simulink model "pompev3"  (R2021a)
settings: Solver=ode15s  StartTime=0.0  StopTime=500.0  FixedStep=0.1  RelTol=1e-3  EnableMultiTasking=on
settings Model: Creator=M1  LastModifiedBy=M1
settings SolverCC: AlgebraicLoopSolver=TrustRegion  AutoInsertRateTranBlk=on
settings DataIOCC: LimitDataPoints=on
settings OptimizationCC: LifeSpan=inf
settings DebuggingCC: AllowSymbolicDim=off  SFUnexpectedBacktrackingDiag=warning  SFNoUnconditionalDefaultTransitionDiag=warning  SFExecutionAtInitializationDiag=none  ArithmeticOperatorsInVariantConditions=warning
settings SFSimCC: SimUseLocalCustomCode=off  CustomCodeUndefinedFunction=UseInterfaceOnly
settings RTWCC: RTWUseLocalCustomCode=off
settings CodeAppCC: StateflowObjectComments=on
settings GRTTargetCC: TargetLangStandard=C89/C90 (ANSI)
settings ConfigComp: CovMetricSettings=dw  CovSaveCumulativeToWorkspaceVar=on  CovSaveSingleToWorkspaceVar=on  CovExternalEMLEnable=off  CovSFcnEnable=off

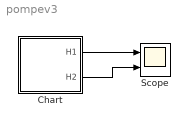
== system pompev3 ==
  Chart : Stateflow chart  TreatAsAtomicUnit=on
  Scope : Scope  NumInputPorts=2
  wires:
  Chart/1(H1) -> Scope/1
  Chart/2(H2) -> Scope/2

== stateflow chart pompev3/Chart ==
  settings: updateMethod=CONTINUOUS
  state Reservoir [parallel]
    settings: executionOrder=1
    state mode_1
      during :
      H1_dot = [(1/S)*(Qp-a*H1(1)^(1/2)-a*sign(H1(1) - H2(1))*abs(H1(1) - H2(1))^(1/2));
      - (2*H1(2))/(385*H1(1)^(1/2)) - (2*sign(H1(1) - H2(1))^2*(H1(2) - H2(2)))/(385*abs(H1(1) - H2(1))^(1/2)) - (8*abs(H1(1) - H2(1))^(1/2)*dirac*(H1(2) - H2(2)))/385];
      H2_dot = [(1/S)*a*sign(H1(1)-H2(1))*abs(H1(1)-H2(1))^(1/2);
      (2*sign(H1(1) - H2(1))^2*(H1(2) - H2(2)))/(385*abs(H1(1) - H2(1))^(1/2)) + (8*abs(H1(1) - H2(1))^(1/2)*dirac*(H1(2) - H2(2)))/385];
    note: modes 1 et 2 sont les états du réservoirs lorsque la vanne V4 est fermée
        | modes 3 et 4 sont les états du réservoirs lorsque la vanne V4 est ouverte
        | les équations se basent sur les écouelemnts de Toricelli
    state mode_2
      during :
      H1_dot = [(1/S)*(Qp-a*H1(1)^(1/2)-a*sign(H1(1) - H2(1))*abs(H1(1) - H2(1))^(1/2)-a*sign(H1(1) - H2(1))*abs(H1(1)-0.5)^(1/2));
      - (2*H1(2))/(385*H1(1)^(1/2)) - (2*sign(H1(1) - H2(1))^2*(H1(2) - H2(2)))/(385*abs(H1(1) - H2(1))^(1/2)) - (8*abs(H1(1) - 1/2)^(1/2)*dirac*(H1(2) - H2(2)))/385- (8*abs(H1(1) - H2(1))^(1/2)*dirac*(H1(2) - H2(2)))/385 - (2*sign(H1(1) - 1/2)*sign(H1(1) - H2(1))*H1(2))/(385*abs(H1(1) - 1/2)^(1/2))];
      H2_dot = [(1/S)*(a*sign(H1(1) - H2(1))*abs(H1(1) - H2(1))^(1/2)+a*sign(H1(1) - H2(1))*abs(H1(1)-0.5)^(1/2));
      (2*sign(H1(1) - H2(1))^2*(H1(2) - H2(2)))/(385*abs(H1(1) - H2(1))^(1/2)) + (8*abs(H1(1) - 1/2)^(1/2)*dirac*(H1(2) - H2(2)))/385+ (8*abs(H1(1) - H2(1))^(1/2)*dirac*(H1(2) - H2(2)))/385 + (2*sign(H1(1) - 1/2)*sign(H1(1) - H2(1))*H1(2))/(385*abs(H1(1) - 1/2)^(1/2))];
    state mode_4
      during :
      H1_dot = [(1/S)*(Qp-a*H1(1)^(1/2)-a*sign(H1(1)-H2(1))*abs(H1(1)-H2(1))^(1/2));
      - (2*H2(2))/(385*H1(1)^(1/2)) - (2*sign(H1(1) - H2(1))^2*(H1(2) - H2(2)))/(385*abs(H1(1) - H2(1))^(1/2)) - (8*abs(H1(1) - H2(1))^(1/2)*dirac*(H1(2) - H2(2)))/385];
      H2_dot = [(1/S)*(a*sign(H1(1) - H2(1))*abs(H1(1) - H2(1))^(1/2)-a*H2(1)^(1/2));
      (2*sign(H1(1) - H2(1))^2*(H1(2) - H2(2)))/(385*abs(H1(1) - H2(1))^(1/2)) - (2*H2(2))/(385*H2(1)^(1/2)) + (8*abs(H1(1) - H2(1))^(1/2)*dirac*(H1(2) - H2(2)))/385];
    state mode_3
      during :
      H1_dot = [(1/S)*(Qp-a*H1(1)^(1/2)-a*sign(H1(1) - H2(1))*abs(H1(1) - H2(1))^(1/2)-a*sign(H1(1) - H2(1))*abs(H1(1)-0.5)^(1/2));
      - (2*H1(2))/(385*H1(1)^(1/2)) - (2*sign(H1(1) - H2(1))^2*(H1(2) - H2(2)))/(385*abs(H1(1) - H2(1))^(1/2)) - (8*abs(H1(1) - 1/2)^(1/2)*dirac*(H1(2) - H2(2)))/385- (8*abs(H1(1) - H2(1))^(1/2)*dirac*(H1(2) - H2(2)))/385 - (2*sign(H1(1) - 1/2)*sign(H1(1) - H2(1))*H1(2))/(385*abs(H1(1) - 1/2)^(1/2))];
      H2_dot = [(1/S)*(a*sign(H1(1) - H2(1))*abs(H1(1) - H2(1))^(1/2) + a*sign(H1(1) - H2(1))*abs(H1(1)-0.5)^(1/2)-a*H2(1)^(1/2));
      (2*sign(H1(1) - H2(1))^2*(H1(2) - H2(2)))/(385*abs(H1(1) - H2(1))^(1/2)) - (2*H2(2))/(385*H2(1)^(1/2)) + (8*abs(H1(1) - 1/2)^(1/2)*dirac*(H1(2) - H2(2)))/385+ (8*abs(H1(1) - H2(1))^(1/2)*dirac*(H1(2) - H2(2)))/385 + (2*sign(H1(1) - 1/2)*sign(H1(1) - H2(1))*H1(2))/(385*abs(H1(1) - 1/2)^(1/2))];
    mode_2 -> mode_1 [order 3] : [H1(1)<=0.5]
    mode_1 -> mode_2 [order 4] : [H1(1) >= 0.5]
    mode_2 -> mode_2 [order 2] : [dirac == 1 && H2(1) ~= H1(1)]{dirac = 0}
    mode_2 -> mode_2 [order 1] : [H1(1)==H2(1)]{dirac = 1}
    mode_4 -> mode_1 [order 3] : [in(Vanne1.ferme)]
    mode_1 -> mode_4 [order 3] : [in(Vanne1.ouvert)]
    mode_1 -> mode_1 [order 1] : [H1(1)==H2(1)]{dirac = 1}
    mode_1 -> mode_1 [order 2] : [dirac == 1 && H2(1) ~= H1(1)]{dirac = 0}
    mode_3 -> mode_2 [order 4] : [in(Vanne1.ferme)]
    mode_2 -> mode_3 [order 4] : [in(Vanne1.ouvert)]
    mode_4 -> mode_4 [order 1] : [H1(1)==H2(1)]{dirac = 1}
    mode_4 -> mode_4 [order 2] : [dirac == 1 && H2(1) ~= H1(1)]{dirac = 0}
    mode_3 -> mode_3 [order 2] : [H1(1)==H2(1)]{dirac = 1}
    mode_3 -> mode_3 [order 1] : [dirac == 1 && H2(1) ~= H1(1)]{dirac = 0}
    mode_3 -> mode_4 [order 3] : [H1(1) <= 0.5]
    mode_4 -> mode_3 [order 4] : [H1(1) >= 0.5]
  state Vanne1 [parallel]
    settings: executionOrder=2
    note: Vanne1 ouvre le conduit V4
        | Vanne 2 le ferme
    state ferme
    state ouvert
    (default) -> ferme
    ouvert -> ferme : [after(140, sec)]
    ferme -> ouvert : [after(240, sec)]
  state Pompe [parallel]
    settings: executionOrder=3
    state En_marche
      during :
      Qp_dot = 0;
    state Arret
      during:
      Qp_dot = 0;
    note: en fonction de différents critères,
        | sur la hauteur du réservoir h2 et
        | la vitesse de h2 on arrête ou allume
        | la pompe
    (default) -> Arret
    En_marche -> Arret : [(H2(1)>0.2)||(H2(1)>0.1&&H2(2)<0)]{Qp = 0}
    Arret -> En_marche : [(H2(1)<0.1)||(H2(1)<0.2&&H2(2)>0)]{Qp = 0.001}
  (default) -> mode_1
  data: Qp local double =0.001; S constant double =0.0154; H1 output size=[2, 1] =[0.4; 0]; H2 output size=[2, 1] =[0; 0]; a constant double =0.00016; dirac local =0
  data Qp settings: updateMethod=SF_CONTINUOUS_TIME_DATA
  data H1 settings: updateMethod=SF_CONTINUOUS_TIME_DATA
  data H2 settings: updateMethod=SF_CONTINUOUS_TIME_DATA
